simulink subsystem "AppliedForceScale"  (R2023a)
settings: Solver=VariableStepAuto  StartTime=0.0  StopTime=10.0  RelTol=1e-3

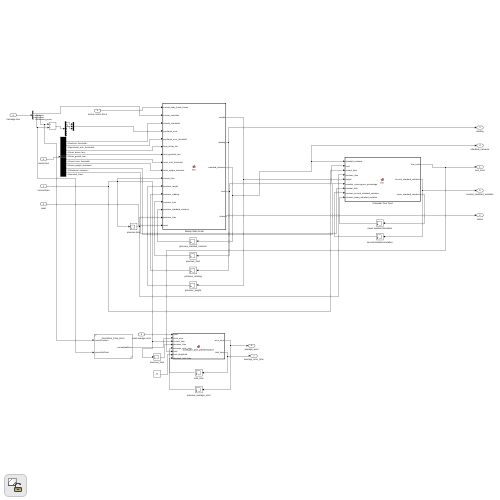
[thumbnail: Simulink's stored preview of the top-level diagram]
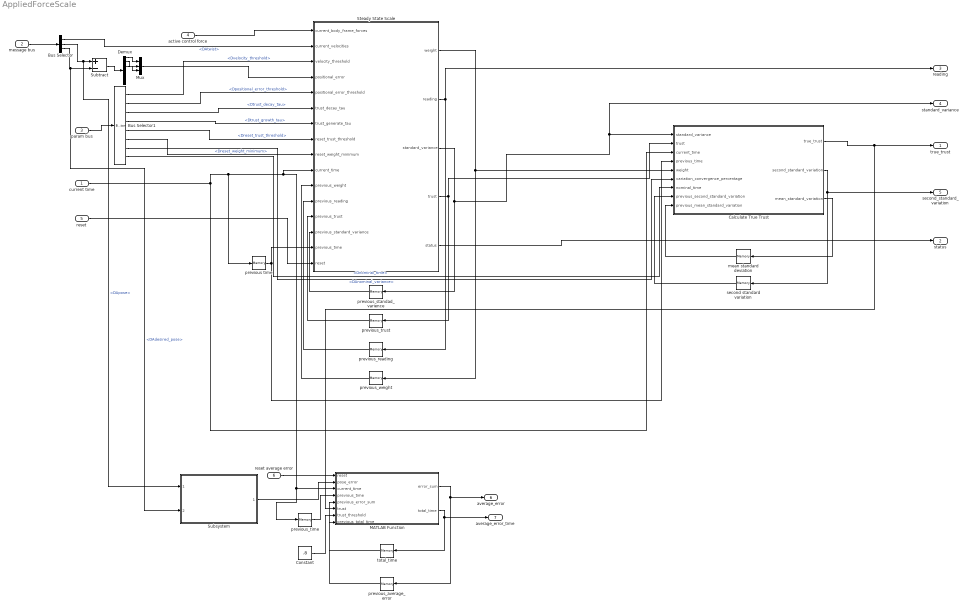
== system AppliedForceScale ==
  current time : Inport
  message bus : Inport  Port=2
  param bus : Inport  Port=3
  active control force : Inport  Port=4
  reset : Inport  Port=5
  reset average error : Inport  Port=6  OutDataTypeStr=boolean
  Bus Selector : BusSelector  OutputSignals=current_state.DAtwist,current_state.DApose,desired_pose.DAdesired_pose
  Bus Selector1 : BusSelector  OutputSignals=Dvelocity_threshold,Dpositional_error_threshold,Dtrust_decay_tau,Dtrust_growth_tau,Dreset_trust_threshold,Dreset_weight_minimum,DAnominal_variance,Dnominal_time
  Calculate True Trust : MATLAB Function  TreatAsAtomicUnit=on
  Constant : Constant  Value=.8
  Demux : Demux  Outputs=7
  MATLAB Function : MATLAB Function  TreatAsAtomicUnit=on
  Mux : Mux  Inputs=3
  Steady State Scale : MATLAB Function  TreatAsAtomicUnit=on
  Subsystem : Subsystem  ReferencedSubsystem=Normalize_Pose_Error
  Subtract : Sum  Inputs=+-
  mean standard deviation : Memory  InitialCondition=[0,0,0,0,0,0]'
  previous time : Memory
  previous_average_error : Memory  InitialCondition=[0;0;0;0;0;0]
  previous_reading : Memory  InitialCondition=[0,0,0,0,0,0]'
  previous_standad_varience : Memory  InitialCondition=[0,0,0,0,0,0]'
  previous_time : Memory  InitialCondition=-1
  previous_trust : Memory
  previous_weight : Memory
  second standard variation : Memory  InitialCondition=[0,0,0,0,0,0]'
  total_time : Memory
  true_trust : Outport
  status : Outport  Port=2
  reading : Outport  Port=3
  standard_variance : Outport  Port=4
  second_standard_variation : Outport  Port=5
  average_error : Outport  Port=6
  average_error_time : Outport  Port=7
  wires:
  Calculate True Trust/1(true_trust) -> true_trust/1, MATLAB Function/6(trust)
  previous_weight/1 -> Steady State Scale/11(previous_weight)
  previous_trust/1 -> Steady State Scale/13(previous_trust)
  previous_reading/1 -> Steady State Scale/12(previous_reading)
  Steady State Scale/1(weight) -> Calculate True Trust/5(weight), previous_weight/1
  Steady State Scale/4(trust) -> Calculate True Trust/2(trust), previous_trust/1
  current time/1 -> Calculate True Trust/3(current_time), previous time/1, Steady State Scale/10(current_time), MATLAB Function/3(current_time), previous_time/1
  Steady State Scale/3(standard_variance) -> Calculate True Trust/1(standard_variance), standard_variance/1, previous_standad_varience/1
  previous_standad_varience/1 -> Steady State Scale/14(previous_standard_variance)
  Steady State Scale/2(reading) -> reading/1, previous_reading/1
  Steady State Scale/5(status) -> status/1
  previous time/1 -> Steady State Scale/15(previous_time), Calculate True Trust/4(previous_time)
  active control force/1 -> Steady State Scale/1(current_body_frame_forces)
  message bus/1 -> Bus Selector/1
  param bus/1 -> Bus Selector1/1
  Bus Selector1/6 -> Steady State Scale/9(reset_weight_minimum)  "<Dreset_weight_minimum>"
  Bus Selector1/5 -> Steady State Scale/8(reset_trust_threshold)  "<Dreset_trust_threshold>"
  Bus Selector1/4 -> Steady State Scale/7(trust_generate_tau)  "<Dtrust_growth_tau>"
  Bus Selector1/2 -> Steady State Scale/5(positional_error_threshold)  "<Dpositional_error_threshold>"
  Bus Selector1/1 -> Steady State Scale/3(velocity_threshold)  "<Dvelocity_threshold>"
  Bus Selector1/3 -> Steady State Scale/6(trust_decay_tau)  "<Dtrust_decay_tau>"
  Bus Selector1/7 -> Calculate True Trust/6(variation_convergence_percentage)  "<DAnominal_variance>"
  Bus Selector/1 -> Steady State Scale/2(current_velocities)  "<DAtwist>"
  Bus Selector/2 -> Subtract/1, Subsystem/1  "<DApose>"
  Bus Selector/3 -> Subtract/2, Subsystem/2  "<DAdesired_pose>"
  Subtract/1 -> Demux/1
  Demux/3 -> Mux/3
  Demux/2 -> Mux/2
  Demux/1 -> Mux/1
  Mux/1 -> Steady State Scale/4(positional_error)
  Calculate True Trust/3(mean_standard_variation) -> mean standard deviation/1
  mean standard deviation/1 -> Calculate True Trust/9(previous_mean_standard_variation)
  Calculate True Trust/2(second_standard_variation) -> second_standard_variation/1, second standard variation/1
  second standard variation/1 -> Calculate True Trust/8(previous_second_standard_variation)
  Bus Selector1/8 -> Calculate True Trust/7(nominal_time)  "<Dnominal_time>"
  reset/1 -> Steady State Scale/16(reset)
  Subsystem/1 -> MATLAB Function/2(pose_error)
  previous_average_error/1 -> MATLAB Function/5(previous_error_sum)
  MATLAB Function/1(error_sum) -> previous_average_error/1, average_error/1
  previous_time/1 -> MATLAB Function/4(previous_time)
  Constant/1 -> MATLAB Function/7(trust_threshold)
  total_time/1 -> MATLAB Function/8(previous_total_time)
  MATLAB Function/2(total_time) -> total_time/1, average_error_time/1
  reset average error/1 -> MATLAB Function/1(reset)

== matlab function AppliedForceScale/Steady State Scale ==
function [weight, reading, standard_variance, trust, status] = fcn(current_body_frame_forces, current_velocities, velocity_threshold, positional_error, positional_error_threshold, trust_decay_tau, trust_generate_tau, reset_trust_threshold, reset_weight_minimum, current_time, previous_weight, previous_reading, previous_trust, previous_standard_variance, previous_time, reset)

%status 
% -10 nans
% -1 discarding measurements
% 0 out of position / velocity threshold
% 1 collecting readings

%if time delta is too large


%readings
reading = previous_reading;
weight = (previous_weight);
standard_variance = previous_standard_variance;

%throw everything out the window if getting nans
if(sum(isnan(weight)) + sum(isnan(reading) + isnan(previous_trust) + sum(isnan(standard_variance)) + sum(isnan(current_body_frame_forces))) > 0)
    weight = 0;
    reading = [0,0,0,0,0,0]';
    trust = 0;
    standard_variance = [0,0,0,0,0,0]';

    status = -10;

    return
end

%throw everything out if FF chnage is applied
if(reset)
    weight = 0;
    reading = [0,0,0,0,0,0]';
    trust = 0;
    standard_variance = [0,0,0,0,0,0]';

    status = -11;

    return
end

if(current_time - previous_time > 1000)
    weight = 0;
    reading = [0,0,0,0,0,0]';
    trust = 0;
    standard_variance = [0,0,0,0,0,0]';

    status = 0;

    return
end

%update time
time = current_time;

%if measurements are trusted
if(norm(current_velocities) < velocity_threshold && norm(positional_error) < positional_error_threshold)

    weight = (previous_weight) + (current_time - previous_time);

    %update readings
    reading = ((previous_reading * previous_weight) + ((current_time - previous_time) * current_body_frame_forces)) / weight;

    %update variance via welford's online algorithm
    standard_variance = previous_standard_variance + ((current_body_frame_forces - reading) .* (current_body_frame_forces - previous_reading) - previous_standard_variance) * (current_time - previous_time) / weight;

    %increase trust as a reading
    trust = 1 - (1 - previous_trust) * exp(-(time - previous_time) / trust_generate_tau);

    status = 1;

else
    
    %decay trust
    trust = previous_trust * exp(-(time - previous_time)/trust_decay_tau);

    status = 0;

end


%if no trust - trash the system and try again
if((trust <  reset_trust_threshold && weight > reset_weight_minimum) || trust == 0 || weight == 0)
    trust = 0;
    weight = 0;
    reading = [0,0,0,0,0,0]';
    standard_variance = [0,0,0,0,0,0]';

    status = -1;
end

== matlab function AppliedForceScale/Calculate True Trust ==
function [true_trust, second_standard_variation, mean_standard_variation] = fcn(standard_variance, trust, current_time, previous_time, weight, variation_convergence_percentage, nominal_time, previous_second_standard_variation, previous_mean_standard_variation)

%calculate trust based on T-Distribution and measurement frequency

true_trust = [0,0,0,0,0,0]';
second_standard_variation = [0,0,0,0,0,0]';
mean_standard_variation = [0,0,0,0,0,0]';

%if the time difference is significant
if(current_time - previous_time > 1000)
    return
end

%standard variance 
if(min(standard_variance) < 0)
    return
end

%if the measurement was reset
if(weight == 0)
    return
end

if(sum(isnan(previous_second_standard_variation)) + sum(isnan(previous_mean_standard_variation)) > 0)
    %return to reset nan condition
    
    return
end

%change in time since last run
delta_T = current_time - previous_time;

%update the mean standard deviation
mean_standard_variation = ((weight - delta_T) * previous_mean_standard_variation + standard_variance * delta_T) / (weight);

%standard variance of the standard variance 
second_standard_variation = previous_second_standard_variation + ((standard_variance - previous_mean_standard_variation).*(standard_variance - mean_standard_variation) - previous_second_standard_variation) / (weight + delta_T);

if(min(second_standard_variation) < 0)
    return
end

%probality that the standard variation has converged to a percentage
%difference
settling_trust = tcdf((variation_convergence_percentage * mean_standard_variation) ./ sqrt(second_standard_variation), weight / nominal_time);

true_trust = settling_trust * trust;

== matlab function AppliedForceScale/MATLAB Function ==
function [error_sum, total_time]  = evaluate_axis_performance(reset, pose_error, current_time, previous_time, previous_error_sum, trust, trust_threshold, previous_total_time)

error_sum = previous_error_sum;
total_time = previous_total_time;

if(previous_time < 0)
    error_sum = [0;0;0;0;0;0];
    total_time = 0;
    return
end

if(reset == true)
    error_sum = [0;0;0;0;0;0];
    total_time = 0;
    return
end

if(max(trust) > trust_threshold)
    error_sum = (previous_error_sum * previous_total_time + abs(pose_error') * (current_time - previous_time)) / ((current_time - previous_time) + previous_total_time);
    total_time = previous_total_time + (current_time - previous_time);
else
    error_sum = [0;0;0;0;0;0];
    total_time = 0;
end
